simulink model "CRFB5"  (R2017a)
settings: Solver=FixedStepAuto  StartTime=0.0  StopTime=10.0  RelTol=1e-3
undefined symbols (not defined in the file): a, b, c, DiscIntNeverNeededParam, g
settings Model: Creator=bhannigan  LastModifiedBy=bhannigan

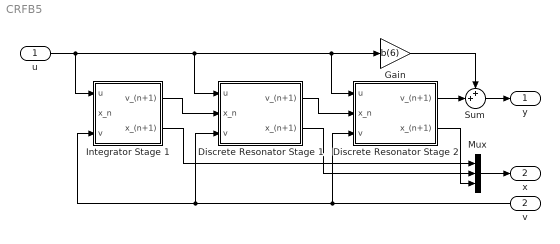
== system CRFB5 ==
  u : Inport
  v : Inport  Port=2
  Discrete Resonator Stage 1 : Subsystem  mask{a_1=a(2), a_2=a(3), b_1=b(2), b_2=b(3), c_1=c(2), c_2=c(3), g=g(1), sat_u=Inf, sat_l=-Inf, t_s=6.25e-6}
      mask prompts: a_1 "Feedback gain n:"; a_2 "Feedback gain n+1:"; b_1 "Feedforward gain n:"; b_2 "Feedforward gain n+1:"; c_1 "Gain n:"; c_2 "Gain n+1:"; g "Internal gain:"; sat_u "Upper limit:"; sat_l "Lower limit:"; t_s "Sample time (-1 for inherited):"
      mask DialogControl Container3 Prompt: Gains
      mask DialogControl Container4 Prompt: State Saturation
  Discrete Resonator Stage 2 : Subsystem  mask{a_1=a(4), a_2=a(5), b_1=b(4), b_2=b(5), c_1=c(4), c_2=c(5), g=g(2), sat_u=Inf, sat_l=-Inf, t_s=6.25e-6}
      mask prompts: a_1 "Feedback gain n:"; a_2 "Feedback gain n+1:"; b_1 "Feedforward gain n:"; b_2 "Feedforward gain n+1:"; c_1 "Gain n:"; c_2 "Gain n+1:"; g "Internal gain:"; sat_u "Upper limit:"; sat_l "Lower limit:"; t_s "Sample time (-1 for inherited):"
      mask DialogControl Container3 Prompt: Gains
      mask DialogControl Container4 Prompt: State Saturation
  Gain : Gain  Gain=b(6)
  Integrator Stage 1 : Subsystem  mask{a=a(1), b=b(1), c=c(1), sat_u=Inf, sat_l=-Inf, t_s=6.25e-6}
      mask prompts: a "Feedback gain:"; b "Feedforward gain:"; c "Gain:"; sat_u "Upper limit:"; sat_l "Lower limit:"; t_s "Sample time (-1 for inherited):"
  Mux : Mux  Inputs=3
  Sum : Sum  Inputs=++|
  y : Outport
  x : Outport  Port=2
  wires:
  Integrator Stage 1/1(v_(n+1)) -> Discrete Resonator Stage 1/2(x_n)
  Discrete Resonator Stage 1/1(v_(n+1)) -> Discrete Resonator Stage 2/2(x_n)
  v/1 -> Discrete Resonator Stage 2/3(v), Discrete Resonator Stage 1/3(v), Integrator Stage 1/3(v)
  Sum/1 -> y/1
  Gain/1 -> Sum/1
  Discrete Resonator Stage 2/1(v_(n+1)) -> Sum/2
  Integrator Stage 1/2(x_(n+1)) -> Mux/1
  Discrete Resonator Stage 1/2(x_(n+1)) -> Mux/2
  Discrete Resonator Stage 2/2(x_(n+1)) -> Mux/3
  Mux/1 -> x/1
  u/1 -> Discrete Resonator Stage 2/1(u), Gain/1, Discrete Resonator Stage 1/1(u), Integrator Stage 1/1(u)

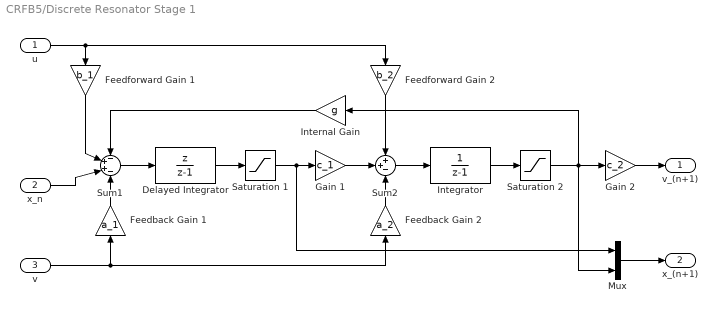
== system CRFB5/Discrete Resonator Stage 1 ==
  u : Inport
  x_n : Inport  Port=2
  v : Inport  Port=3
  Delayed Integrator : DiscreteTransferFcn  Numerator=[1 0]  Denominator=[1 -1]  SampleTime=t_s
  Feedback Gain 1 : Gain  Gain=a_1
  Feedback Gain 2 : Gain  Gain=a_2
  Feedforward Gain 1 : Gain  Gain=b_1
  Feedforward Gain 2 : Gain  Gain=b_2
  Gain 1 : Gain  Gain=c_1
  Gain 2 : Gain  Gain=c_2
  Integrator : DiscreteTransferFcn  Denominator=[1 -1]  SampleTime=t_s
  Internal Gain : Gain  Gain=g
  Mux : Mux  Inputs=2
  Saturation 1 : Saturate  UpperLimit=sat_u  LowerLimit=sat_l
  Saturation 2 : Saturate  UpperLimit=sat_u  LowerLimit=sat_l
  Sum1 : Sum  Inputs=-++-
  Sum2 : Sum  Inputs=++-
  v_(n+1) : Outport
  x_(n+1) : Outport  Port=2
  wires:
  Gain 1/1 -> Sum2/2
  Integrator/1 -> Saturation 2/1
  Sum1/1 -> Delayed Integrator/1
  Delayed Integrator/1 -> Saturation 1/1
  Internal Gain/1 -> Sum1/1
  Feedback Gain 1/1 -> Sum1/4
  Feedforward Gain 2/1 -> Sum2/1
  Sum2/1 -> Integrator/1
  x_n/1 -> Sum1/3
  Feedforward Gain 1/1 -> Sum1/2
  v/1 -> Feedback Gain 2/1, Feedback Gain 1/1
  Feedback Gain 2/1 -> Sum2/3
  u/1 -> Feedforward Gain 1/1, Feedforward Gain 2/1
  Gain 2/1 -> v_(n+1)/1
  Mux/1 -> x_(n+1)/1
  Saturation 1/1 -> Mux/1, Gain 1/1
  Saturation 2/1 -> Internal Gain/1, Mux/2, Gain 2/1

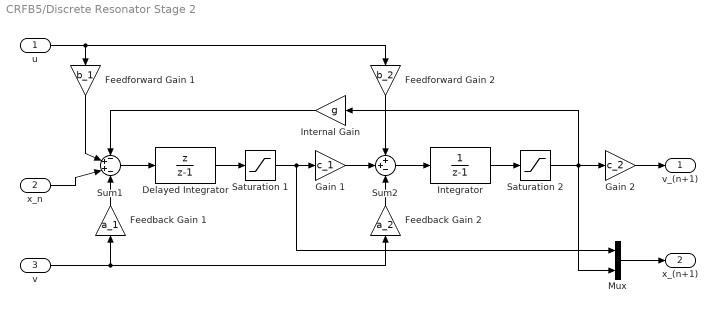
== system CRFB5/Discrete Resonator Stage 2 ==
  u : Inport
  x_n : Inport  Port=2
  v : Inport  Port=3
  Delayed Integrator : DiscreteTransferFcn  Numerator=[1 0]  Denominator=[1 -1]  SampleTime=t_s
  Feedback Gain 1 : Gain  Gain=a_1
  Feedback Gain 2 : Gain  Gain=a_2
  Feedforward Gain 1 : Gain  Gain=b_1
  Feedforward Gain 2 : Gain  Gain=b_2
  Gain 1 : Gain  Gain=c_1
  Gain 2 : Gain  Gain=c_2
  Integrator : DiscreteTransferFcn  Denominator=[1 -1]  SampleTime=t_s
  Internal Gain : Gain  Gain=g
  Mux : Mux  Inputs=2
  Saturation 1 : Saturate  UpperLimit=sat_u  LowerLimit=sat_l
  Saturation 2 : Saturate  UpperLimit=sat_u  LowerLimit=sat_l
  Sum1 : Sum  Inputs=-++-
  Sum2 : Sum  Inputs=++-
  v_(n+1) : Outport
  x_(n+1) : Outport  Port=2
  wires:
  Gain 1/1 -> Sum2/2
  Integrator/1 -> Saturation 2/1
  Sum1/1 -> Delayed Integrator/1
  Delayed Integrator/1 -> Saturation 1/1
  Internal Gain/1 -> Sum1/1
  Feedback Gain 1/1 -> Sum1/4
  Feedforward Gain 2/1 -> Sum2/1
  Sum2/1 -> Integrator/1
  x_n/1 -> Sum1/3
  Feedforward Gain 1/1 -> Sum1/2
  v/1 -> Feedback Gain 2/1, Feedback Gain 1/1
  Feedback Gain 2/1 -> Sum2/3
  u/1 -> Feedforward Gain 1/1, Feedforward Gain 2/1
  Gain 2/1 -> v_(n+1)/1
  Mux/1 -> x_(n+1)/1
  Saturation 1/1 -> Mux/1, Gain 1/1
  Saturation 2/1 -> Internal Gain/1, Mux/2, Gain 2/1

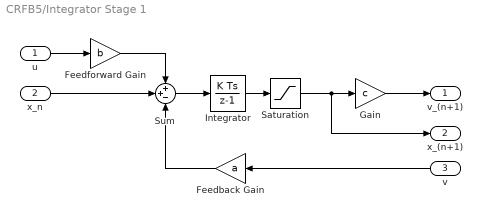
== system CRFB5/Integrator Stage 1 ==
  u : Inport
  x_n : Inport  Port=2
  v : Inport  Port=3
  Feedback Gain : Gain  Gain=a
  Feedforward Gain : Gain  Gain=b
  Gain : Gain  Gain=c
  Integrator : DiscreteIntegrator  InitialConditionSetting=State (most efficient)  SampleTime=t_s  LimitOutput=on  UpperSaturationLimit=Inf  LowerSaturationLimit=-Inf  ICPrevOutput=DiscIntNeverNeededParam  ICPrevScaledInput=DiscIntNeverNeededParam
  Saturation : Saturate  UpperLimit=sat_u  LowerLimit=sat_l
  Sum : Sum  Inputs=++-
  v_(n+1) : Outport
  x_(n+1) : Outport  Port=2
  wires:
  v/1 -> Feedback Gain/1
  Integrator/1 -> Saturation/1
  u/1 -> Feedforward Gain/1
  Feedforward Gain/1 -> Sum/1
  Feedback Gain/1 -> Sum/3
  Sum/1 -> Integrator/1
  x_n/1 -> Sum/2
  Gain/1 -> v_(n+1)/1
  Saturation/1 -> x_(n+1)/1, Gain/1
